simulink model "SSB_LC"  (R2024a)
settings: Solver=VariableStepAuto  StartTime=0.0  StopTime=10.0  RelTol=1e-3
libraries: dspfdesign x1
settings Model: Creator=mohamed
settings SolverCC: AlgebraicLoopSolver=TrustRegion
settings DebuggingCC: UnconnectedInputMsg=warning  UnconnectedOutputMsg=warning  UnconnectedLineMsg=warning
settings ModelReferenceCC: EnableRefExpFcnMdlSchedulingChecks=on
settings SFSimCC: CustomCodeUndefinedFunction=UseInterfaceOnly
settings RTWCC: GPUComputeCapability=3.5  DLArmComputeVersion=19.05

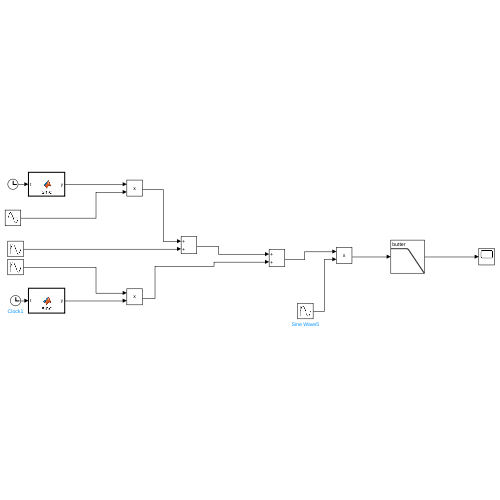
[thumbnail: Simulink's stored preview of the top-level diagram]
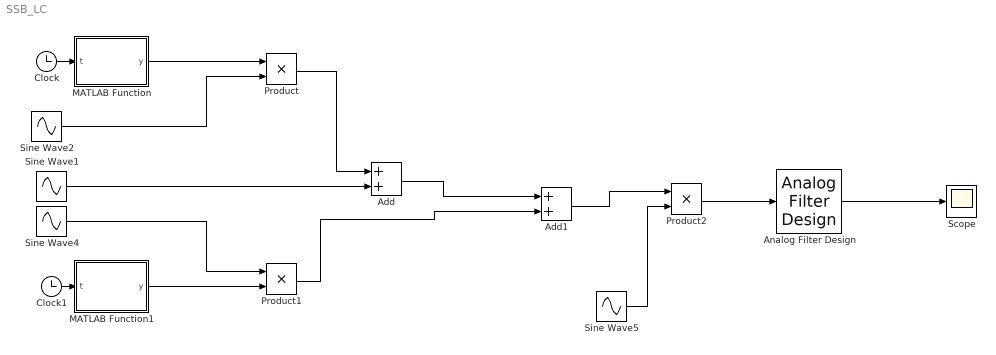
== system SSB_LC ==
  Add : Sum
  Add1 : Sum
  Analog Filter Design : dspfdesign/Analog Filter Design  method=Butterworth  filttype=Lowpass  N=8  Wlo=10*pi  Whi=80  Rp=2  Rs=40
  Clock : Clock
      settings: Decimation=500
  Clock1 : Clock
      settings: Decimation=500
  MATLAB Function : MATLAB Function  TreatAsAtomicUnit=on
  MATLAB Function1 : MATLAB Function  TreatAsAtomicUnit=on
  Product : Product
  Product1 : Product
  Product2 : Product
  Scope : Scope
  Sine Wave1 : Sin  Frequency=2000*pi  Phase=pi/2  SampleTime=0
  Sine Wave2 : Sin  Frequency=2000*pi  Phase=pi/2  SampleTime=0
  Sine Wave4 : Sin  Frequency=2000*pi  SampleTime=0
  Sine Wave5 : Sin  Frequency=2000*pi  Phase=pi/2  SampleTime=0
  wires:
  Sine Wave1/1 -> Add/2
  Product/1 -> Add/1
  Sine Wave4/1 -> Product1/1
  Sine Wave5/1 -> Product2/2
  Product2/1 -> Analog Filter Design/1
  Analog Filter Design/1 -> Scope/1
  Product1/1 -> Add1/2
  Clock/1 -> MATLAB Function/1(t)
  Add/1 -> Add1/1
  Clock1/1 -> MATLAB Function1/1(t)
  Add1/1 -> Product2/1
  MATLAB Function1/1(y) -> Product1/2
  Sine Wave2/1 -> Product/2
  MATLAB Function/1(y) -> Product/1

== matlab function SSB_LC/MATLAB Function1 ==
  data: y output; t input
function y = sinc(t)
y = (sinc(5*pi()*t)^2)*(5*pi()*t);

== matlab function SSB_LC/MATLAB Function ==
  data: y output; t input
function y = sinc(t)
y = sinc(10*pi()*t);
